simulink model "Observer_load_torque"  (R2016b)
settings: Solver=FixedStepAuto  StartTime=0.0  StopTime=5  FixedStep=0.00001  RelTol=1e-3
settings Model: Creator=emilio  LastModifiedBy=danielesmn

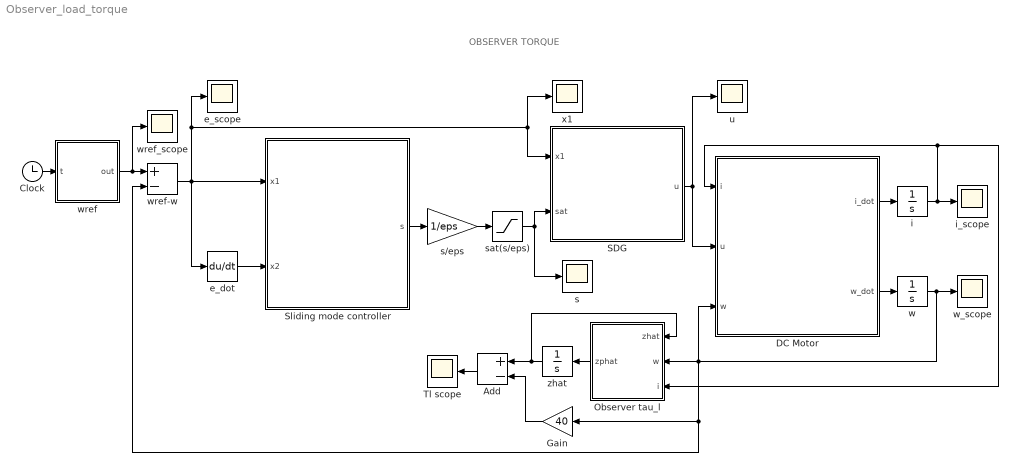
== system Observer_load_torque ==
  note: OBSERVER TORQUE
  Add : Sum  Inputs=+-
  Clock : Clock
  DC Motor : MATLAB Function  TreatAsAtomicUnit=on
  Gain : Gain  Gain=40
  Observer tau_l : MATLAB Function  TreatAsAtomicUnit=on
  SDG : MATLAB Function  TreatAsAtomicUnit=on
  Sliding mode controller : MATLAB Function  TreatAsAtomicUnit=on
  Tl scope : Scope
  e_dot : Derivative
  e_scope : Scope
  i : Integrator
  i_scope : Scope
  s : Scope
  s/eps : Gain  Gain=1/eps
  sat(s/eps) : Saturate  UpperLimit=1  LowerLimit=-1  ZeroCross=off
  u : Scope
  w : Integrator
  w_scope : Scope
  wref : MATLAB Function  TreatAsAtomicUnit=on
  wref-w : Sum  Inputs=+-
  wref_scope : Scope
  x1 : Scope
  zhat : Integrator  InitialCondition=0.1
  wires:
  wref-w/1 -> e_scope/1, x1/1, SDG/1(x1), Sliding mode controller/1(x1), e_dot/1
  wref/1(out) -> wref_scope/1, wref-w/1
  e_dot/1 -> Sliding mode controller/2(x2)
  Clock/1 -> wref/1(t)
  DC Motor/1(i_dot) -> i/1
  DC Motor/2(w_dot) -> w/1
  w/1 -> wref-w/2, Gain/1, DC Motor/3(w), Observer tau_l/2(w), w_scope/1
  i/1 -> i_scope/1, Observer tau_l/3(i), DC Motor/1(i)
  s/eps/1 -> sat(s/eps)/1
  Sliding mode controller/1(s) -> s/eps/1
  SDG/1(u) -> u/1, DC Motor/2(u)
  sat(s/eps)/1 -> SDG/2(sat), s/1
  Observer tau_l/1(zphat) -> zhat/1
  zhat/1 -> Add/1, Observer tau_l/1(zhat)
  Add/1 -> Tl scope/1
  Gain/1 -> Add/2

== matlab function Observer_load_torque/SDG ==
  data: x1 input; u output; sat input
function u = StateDependentGain(x1, sat)

u0 = 1;
delta = 10;

u = (u0 + delta*abs(x1))*sat;

== matlab function Observer_load_torque/Sliding mode controller ==
  data: x1 input; x2 input; s output
function s = SMC(x1, x2)

c = 30;

s = c*x1 + x2;

== matlab function Observer_load_torque/Observer tau_l ==
  data: zhat input; zphat output; w input; i input
function zphat = ObserverTl(zhat, w, i)

J = 0.001; % kg*m^2
kt = 0.008; % N*m/A
l = 40;

zphat = 1/J*(-l*zhat + l^2*w + l*kt*i);

== matlab function Observer_load_torque/wref ==
  data: t input; out output
function out = input(t)

if t > 2 && t < 3.5
    out = 1;
else
    out = -1;
end

== matlab function Observer_load_torque/DC Motor ==
  data: i input; i_dot output; u input; w input; w_dot output
function [i_dot, w_dot] = Dc_Motor(i, u, w) % i: armature current w: shaft speed

%% Model of the DC Motor

L = 0.001;        %Armature inductance (H)
R = 0.5;          %Armature resistance (Ohm)
kt = 0.008;       %Torque constant (Nm/A)
J = 0.001;        %Inertia of the motor rotor (Kg*m^2)
B = 0.01;         %Coefficient of viscous friction (Nm*s/rad)
lambda0 = 0.001;  %Back electromotive force (EMF) constant (V*s/rad)

tauL = B*w;        %Load torque

i_dot = u/L - R/L*i - lambda0/L*w;      %Electrical part model
w_dot = (kt*i - tauL)/J;              %Mechanical part model
